simulink model "EngineBleedAirSystem"  (R2018b)
settings: Solver=FixedStepAuto  StartTime=0.0  StopTime=500  FixedStep=0.01  RelTol=1e-3
values from neighbouring files (symbols this model uses):
  AirSourceMode = 2    [run_sim.m]
libraries: simulink x2
settings Model: Creator=ZhaoJiance  LastModifiedBy=ZhaoJiance

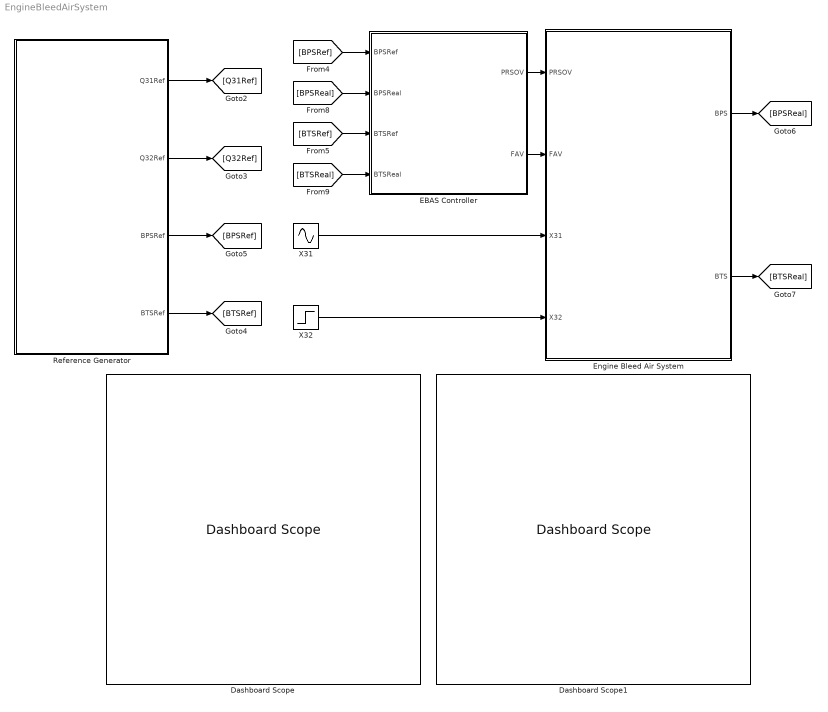
== system EngineBleedAirSystem ==
  Dashboard Scope : DashboardScope  WebBlockId=85
  Dashboard Scope1 : DashboardScope  WebBlockId=86
  EBAS Controller : Subsystem  VariantControlMode=Label  Variant=on  VariantControl=Variant1  LabelModeActiveChoice=L1AC
  Engine Bleed Air System : Subsystem
  Reference Generator : Subsystem
  X31 : Sin  Amplitude=10  Bias=50  Frequency=0.1  SampleTime=0
  X32 : Step  Time=0  Before=50  After=30  SampleTime=0
  wires:
  [BTSRef] -> EBAS Controller/3("BTSRef  ")
  [BPSReal] -> EBAS Controller/2("BPSReal ")
  EBAS Controller/2(" FAV") -> Engine Bleed Air System/2(FAV)
  Engine Bleed Air System/2(BTS) -> [BTSReal]
  Engine Bleed Air System/1(BPS) -> [BPSReal]
  EBAS Controller/1(" PRSOV") -> Engine Bleed Air System/1(PRSOV)
  [BPSRef] -> EBAS Controller/1("BPSRef  ")
  X31/1 -> Engine Bleed Air System/3(X31)
  [BTSReal] -> EBAS Controller/4("BTSReal  ")
  Reference Generator/4(BTSRef) -> [BTSRef]
  Reference Generator/2(Q32Ref) -> [Q32Ref]
  Reference Generator/1(Q31Ref) -> [Q31Ref]
  Reference Generator/3(BPSRef) -> [BPSRef]
  X32/1 -> Engine Bleed Air System/4(X32)

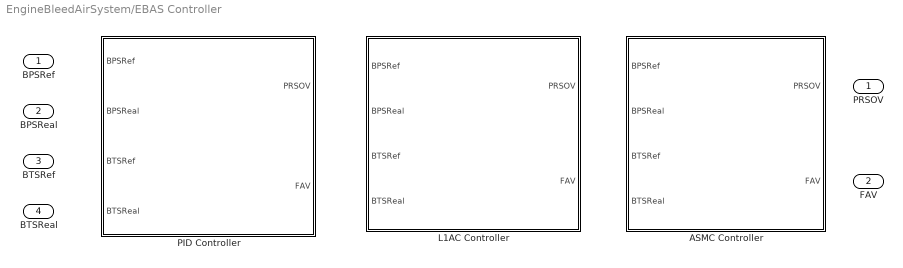
== system EngineBleedAirSystem/EBAS Controller ==
  "BPSRef  " : Inport
  "BPSReal " : Inport  Port=2
  "BTSRef  " : Inport  Port=3
  "BTSReal  " : Inport  Port=4
  ASMC Controller : Subsystem  VariantControl=ASMC
  L1AC Controller : Subsystem  VariantControl=L1AC
  PID Controller : Subsystem  VariantControl=PID
  " PRSOV" : Outport
  " FAV" : Outport  Port=2

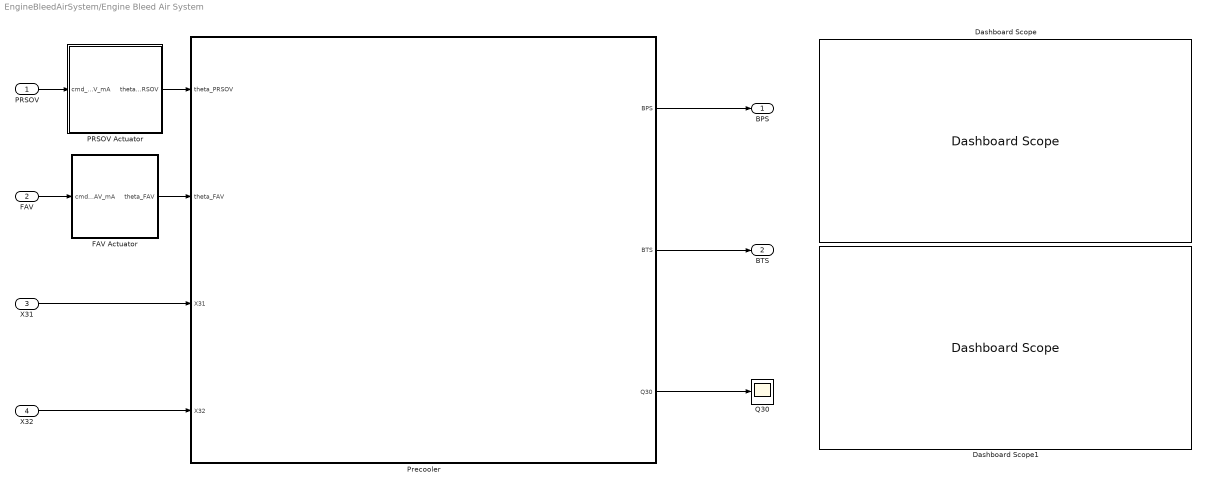
== system EngineBleedAirSystem/Engine Bleed Air System ==
  PRSOV : Inport
  FAV : Inport  Port=2
  X31 : Inport  Port=3
  X32 : Inport  Port=4
  Dashboard Scope : DashboardScope  WebBlockId=89
  Dashboard Scope1 : DashboardScope  WebBlockId=90
  FAV Actuator : MATLAB Function  TreatAsAtomicUnit=on  SystemSampleTime=0.01
  PRSOV Actuator : MATLAB Function  TreatAsAtomicUnit=on  SystemSampleTime=0.01
  Precooler : Subsystem
      mask Display: image('C:\Users\ZhaoJiance\Documents\Github\AeroBleedSimulation\SysID\figure\Precooler.png');
  Q30 : Scope
  BPS : Outport
  BTS : Outport  Port=2
  wires:
  FAV/1 -> FAV Actuator/1(cmd_FAV_mA)
  PRSOV/1 -> PRSOV Actuator/1(cmd_PRSOV_mA)
  PRSOV Actuator/1(theta_PRSOV) -> Precooler/1(theta_PRSOV)
  FAV Actuator/1(theta_FAV) -> Precooler/2(theta_FAV)
  Precooler/1(BPS) -> BPS/1
  Precooler/2(BTS) -> BTS/1
  Precooler/3(Q30) -> Q30/1
  X31/1 -> Precooler/3(X31)
  X32/1 -> Precooler/4(X32)

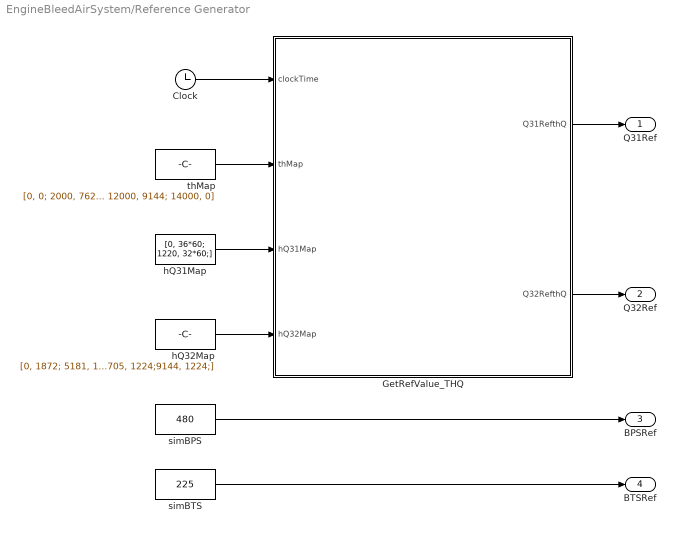
== system EngineBleedAirSystem/Reference Generator ==
  Clock : Clock
  GetRefValue_THQ : MATLAB Function  TreatAsAtomicUnit=on
  hQ31Map : Constant  Value=[0, 36*60; 1220, 32*60;]
  hQ32Map : Constant  Value=[0, 1872; 5181, 1872; 6705, 1224;9144, 1224;]
  simBPS : Constant  Value=480
  simBTS : Constant  Value=225
  thMap : Constant  Value=[0, 0; 2000, 7620; 4000, 7620;6000, 12192; 8000, 12192; 10000, 9144; 12000, 9144; 14000, 0]
  Q31Ref : Outport
  Q32Ref : Outport  Port=2
  BPSRef : Outport  Port=3
  BTSRef : Outport  Port=4
  wires:
  Clock/1 -> GetRefValue_THQ/1(clockTime)
  thMap/1 -> GetRefValue_THQ/2(thMap)
  hQ31Map/1 -> GetRefValue_THQ/3(hQ31Map)
  GetRefValue_THQ/1(Q31RefthQ) -> Q31Ref/1
  hQ32Map/1 -> GetRefValue_THQ/4(hQ32Map)
  GetRefValue_THQ/2(Q32RefthQ) -> Q32Ref/1
  simBTS/1 -> BTSRef/1
  simBPS/1 -> BPSRef/1

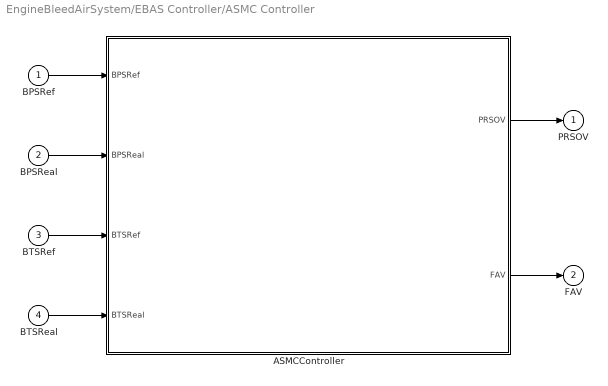
== system EngineBleedAirSystem/EBAS Controller/ASMC Controller ==
  "BPSRef  " : Inport
  "BPSReal " : Inport  Port=2
  "BTSRef  " : Inport  Port=3
  "BTSReal  " : Inport  Port=4
  ASMCController : MATLAB Function  TreatAsAtomicUnit=on  SystemSampleTime=0.01
  " PRSOV" : Outport
  " FAV" : Outport  Port=2
  wires:
  ASMCController/1(PRSOV) -> " PRSOV"/1
  ASMCController/2(FAV) -> " FAV"/1
  "BPSRef  "/1 -> ASMCController/1(BPSRef)
  "BPSReal "/1 -> ASMCController/2(BPSReal)
  "BTSRef  "/1 -> ASMCController/3(BTSRef)
  "BTSReal  "/1 -> ASMCController/4(BTSReal)

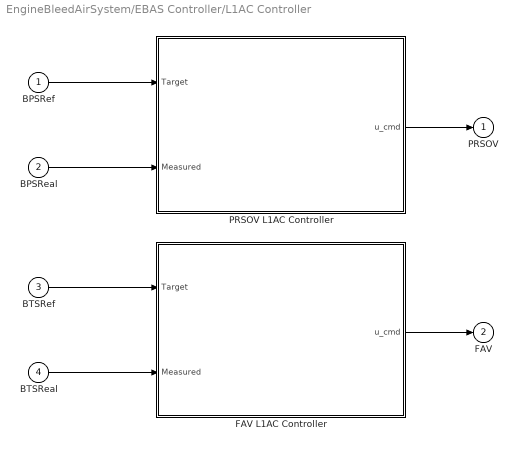
== system EngineBleedAirSystem/EBAS Controller/L1AC Controller ==
  "BPSRef  " : Inport
  "BPSReal " : Inport  Port=2
  "BTSRef  " : Inport  Port=3
  "BTSReal  " : Inport  Port=4
  FAV L1AC Controller : MATLAB Function  TreatAsAtomicUnit=on
  PRSOV L1AC Controller : MATLAB Function  TreatAsAtomicUnit=on
  " PRSOV" : Outport
  " FAV" : Outport  Port=2
  wires:
  FAV L1AC Controller/1(u_cmd) -> " FAV"/1
  PRSOV L1AC Controller/1(u_cmd) -> " PRSOV"/1
  "BPSRef  "/1 -> PRSOV L1AC Controller/1(Target)
  "BPSReal "/1 -> PRSOV L1AC Controller/2(Measured)
  "BTSReal  "/1 -> FAV L1AC Controller/2(Measured)
  "BTSRef  "/1 -> FAV L1AC Controller/1(Target)

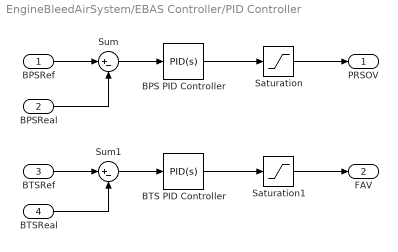
== system EngineBleedAirSystem/EBAS Controller/PID Controller ==
  "BPSRef " : Inport
  BPSReal : Inport  Port=2
  "BTSRef " : Inport  Port=3
  "BTSReal " : Inport  Port=4
  BPS PID Controller : simulink/Continuous/PID Controller  Controller=PID  Form=Parallel  TimeDomain=Continuous-time  SampleTime=-1  IntegratorMethod=Forward Euler  FilterMethod=Forward Euler  ControllerParametersSource=internal  P=0.1  I=0.2  D=0.01  UseFilter=on  N=100  TunerSelectOption=Transfer Function Based (PID Tuner App)  InitialConditionSource=internal  InitialConditionForIntegrator=0  InitialConditionForFilter=0  DifferentiatorICPrevScaledInput=0  ExternalReset=none  TrackingMode=off  Kt=1  LimitOutput=off  UpperSaturationLimit=inf  LowerSaturationLimit=-inf  LinearizeAsGain=on  AntiWindupMode=none  Kb=1  POutMin=[]  POutMax=[]  IOutMin=[]  IOutMax=[]  DOutMin=[]  DOutMax=[]  NOutMin=[]  NOutMax=[]  SumOutMin=[]  SumOutMax=[]  SaturationOutMin=[]  SaturationOutMax=[]  PParamMin=[]  PParamMax=[]  IParamMin=[]  IParamMax=[]  DParamMin=[]  DParamMax=[]  NParamMin=[]  NParamMax=[]  KbParamMin=[]  KbParamMax=[]  KtParamMin=[]  KtParamMax=[]  KbOutMin=[]  KbOutMax=[]  KtOutMin=[]  KtOutMax=[]  IntegratorOutMin=[]  IntegratorOutMax=[]  FilterOutMin=[]  FilterOutMax=[]  SumI1OutMin=[]  SumI1OutMax=[]  SumI2OutMin=[]  SumI2OutMax=[]  SumI3OutMin=[]  SumI3OutMax=[]  SumI4OutMin=[]  SumI4OutMax=[]  SumDOutMin=[]  SumDOutMax=[]  DifferentiatorOutMin=[]  DifferentiatorOutMax=[]  FilterDiffOutCoefMin=[]  FilterDiffOutCoefMax=[]  ReciprocalOutMin=[]  ReciprocalOutMax=[]  SumDenOutMin=[]  SumDenOutMax=[]  SumNumOutMin=[]  SumNumOutMax=[]  DivideOutMin=[]  DivideOutMax=[]  IntegratorContinuousStateAttributes=''  IntegratorStateMustResolveToSignalObject=off  IntegratorRTWStateStorageClass=Auto  FilterContinuousStateAttributes=''  FilterStateMustResolveToSignalObject=off  FilterRTWStateStorageClass=Auto  ParallelPVariant=InternalParameters  IdealPVariant=Disabled  IVariant=InternalParameters  DVariant=InternalParameters  IntegratorVariant=Continuous  SatVariant=Disabled  AWVariant=Passthrough  PCopyVariant=Disabled  TRVariant=Disabled  FdbkBlocksVariant=Forward  IdealPFdbkVariant=Disabled  SatFdbkVariant=Disabled  DerivativeFilterVariant=ContFilter  NVariant=InternalParameters  NCopyVariant=Disabled  FilterICVariant=InternalICsFilter  IntegratorICVariant=InternalICs  ExternalResetVariant=Disabled  TRSumVariant=Passthrough  SumFdbkVariant=Disabled  SumVariant=Sum_PID
  BTS PID Controller : simulink/Continuous/PID Controller  Controller=PID  Form=Parallel  TimeDomain=Continuous-time  SampleTime=-1  IntegratorMethod=Forward Euler  FilterMethod=Forward Euler  ControllerParametersSource=internal  P=-0.1  I=-0.15  D=0  UseFilter=on  N=100  TunerSelectOption=Transfer Function Based (PID Tuner App)  InitialConditionSource=internal  InitialConditionForIntegrator=0  InitialConditionForFilter=0  DifferentiatorICPrevScaledInput=0  ExternalReset=none  TrackingMode=off  Kt=1  LimitOutput=off  UpperSaturationLimit=inf  LowerSaturationLimit=-inf  LinearizeAsGain=on  AntiWindupMode=none  Kb=1  POutMin=[]  POutMax=[]  IOutMin=[]  IOutMax=[]  DOutMin=[]  DOutMax=[]  NOutMin=[]  NOutMax=[]  SumOutMin=[]  SumOutMax=[]  SaturationOutMin=[]  SaturationOutMax=[]  PParamMin=[]  PParamMax=[]  IParamMin=[]  IParamMax=[]  DParamMin=[]  DParamMax=[]  NParamMin=[]  NParamMax=[]  KbParamMin=[]  KbParamMax=[]  KtParamMin=[]  KtParamMax=[]  KbOutMin=[]  KbOutMax=[]  KtOutMin=[]  KtOutMax=[]  IntegratorOutMin=[]  IntegratorOutMax=[]  FilterOutMin=[]  FilterOutMax=[]  SumI1OutMin=[]  SumI1OutMax=[]  SumI2OutMin=[]  SumI2OutMax=[]  SumI3OutMin=[]  SumI3OutMax=[]  SumI4OutMin=[]  SumI4OutMax=[]  SumDOutMin=[]  SumDOutMax=[]  DifferentiatorOutMin=[]  DifferentiatorOutMax=[]  FilterDiffOutCoefMin=[]  FilterDiffOutCoefMax=[]  ReciprocalOutMin=[]  ReciprocalOutMax=[]  SumDenOutMin=[]  SumDenOutMax=[]  SumNumOutMin=[]  SumNumOutMax=[]  DivideOutMin=[]  DivideOutMax=[]  IntegratorContinuousStateAttributes=''  IntegratorStateMustResolveToSignalObject=off  IntegratorRTWStateStorageClass=Auto  FilterContinuousStateAttributes=''  FilterStateMustResolveToSignalObject=off  FilterRTWStateStorageClass=Auto  ParallelPVariant=InternalParameters  IdealPVariant=Disabled  IVariant=InternalParameters  DVariant=InternalParameters  IntegratorVariant=Continuous  SatVariant=Disabled  AWVariant=Passthrough  PCopyVariant=Disabled  TRVariant=Disabled  FdbkBlocksVariant=Forward  IdealPFdbkVariant=Disabled  SatFdbkVariant=Disabled  DerivativeFilterVariant=ContFilter  NVariant=InternalParameters  NCopyVariant=Disabled  FilterICVariant=InternalICsFilter  IntegratorICVariant=InternalICs  ExternalResetVariant=Disabled  TRSumVariant=Passthrough  SumFdbkVariant=Disabled  SumVariant=Sum_PID
  Saturation : Saturate  UpperLimit=400  LowerLimit=0
  Saturation1 : Saturate  UpperLimit=350  LowerLimit=0
  Sum : Sum  Inputs=|+-
  Sum1 : Sum  Inputs=|+-
  PRSOV : Outport
  FAV : Outport  Port=2
  wires:
  Sum1/1 -> BTS PID Controller/1
  BPS PID Controller/1 -> Saturation/1
  BTS PID Controller/1 -> Saturation1/1
  Sum/1 -> BPS PID Controller/1
  BPSReal/1 -> Sum/2
  "BPSRef "/1 -> Sum/1
  "BTSReal "/1 -> Sum1/2
  "BTSRef "/1 -> Sum1/1
  Saturation/1 -> PRSOV/1
  Saturation1/1 -> FAV/1

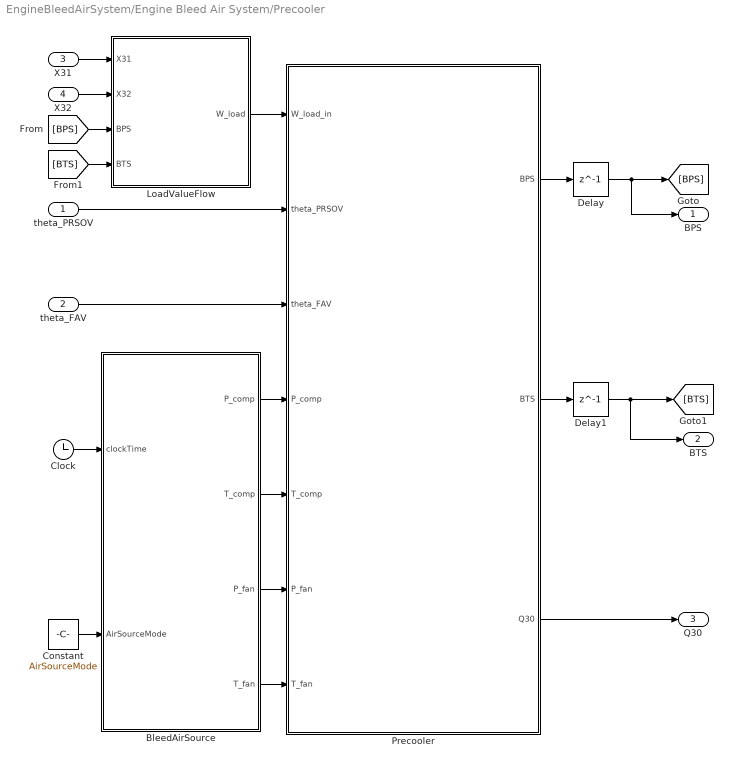
== system EngineBleedAirSystem/Engine Bleed Air System/Precooler ==
  theta_PRSOV : Inport
  theta_FAV : Inport  Port=2
  X31 : Inport  Port=3
  X32 : Inport  Port=4
  BleedAirSource : MATLAB Function  TreatAsAtomicUnit=on  SystemSampleTime=0.01
  Clock : Clock
  Constant : Constant  Value=AirSourceMode
  Delay : Delay  DelayLength=1  InitialCondition=0
  Delay1 : Delay  DelayLength=1  InitialCondition=0
  LoadValueFlow : MATLAB Function  TreatAsAtomicUnit=on  SystemSampleTime=0.01
  Precooler : MATLAB Function  TreatAsAtomicUnit=on  SystemSampleTime=0.01
  BPS : Outport
  BTS : Outport  Port=2
  Q30 : Outport  Port=3
  wires:
  Delay/1 -> BPS/1, [BPS]
  Delay1/1 -> BTS/1, [BTS]
  LoadValueFlow/1(W_load) -> Precooler/1(W_load_in)
  Precooler/1(BPS) -> Delay/1
  Precooler/2(BTS) -> Delay1/1
  Precooler/3(Q30) -> Q30/1
  theta_PRSOV/1 -> Precooler/2(theta_PRSOV)
  theta_FAV/1 -> Precooler/3(theta_FAV)
  X31/1 -> LoadValueFlow/1(X31)
  X32/1 -> LoadValueFlow/2(X32)
  Clock/1 -> BleedAirSource/1(clockTime)
  [BTS] -> LoadValueFlow/4(BTS)
  [BPS] -> LoadValueFlow/3(BPS)
  BleedAirSource/1(P_comp) -> Precooler/4(P_comp)
  BleedAirSource/2(T_comp) -> Precooler/5(T_comp)
  BleedAirSource/3(P_fan) -> Precooler/6(P_fan)
  BleedAirSource/4(T_fan) -> Precooler/7(T_fan)
  Constant/1 -> BleedAirSource/2(AirSourceMode)

== matlab function EngineBleedAirSystem/EBAS Controller/ASMC Controller/ASMCController ==
  data: BPSRef input; PRSOV output; BPSReal input; BTSRef input; BTSReal input; FAV output
function [PRSOV, FAV] = ASMCController(BPSRef, BPSReal, BTSRef, BTSReal)
    % =========================================================================
    % 引气系统控制器 (ESO + ASMC + 逆迟滞补偿)
    %
    % 架构说明:
    %   1. 观测层 (ESO): 实时估计系统内部状态和未知负载扰动(Total Disturbance)。
    %   2. 决策层 (ASMC): 基于扰动补偿的自适应滑模控制，计算理想阀门角度。
    %   3. 补偿层 (Inverse Hys): 将理想角度映射为电流，抵消物理迟滞。
    %
    % 输入:
    %   BPSRef/Real : 压力期望/反馈 [kPa]
    %   BTSRef/Real : 温度期望/反馈 [degC]
    % 输出:
    %   PRSOV    : 热路阀电流 [0-400mA]
    %   FAV      : 冷路阀电流 [0-350mA]
    % =========================================================================

    % --- 1. 系统参数与状态存储 ---
    persistent z1_p z2_p        % 压力ESO状态: z1(压力估计), z2(总扰动)
    persistent z1_t z2_t        % 温度ESO状态: z1(温度估计), z2(总扰动)
    persistent k_asmc_p         % 压力控制器自适应增益
    persistent k_asmc_t         % 温度控制器自适应增益
    persistent last_theta_p     % 上一时刻压力阀角度(用于判断方向)
    persistent last_theta_f     % 上一时刻温度阀角度
    persistent is_init          % 初始化标志

    % --- 2. 参数初始化 ---
    if isempty(is_init)
        % ESO 初始状态
        z1_p = BPSReal; z2_p = 0;
        z1_t = BTSReal; z2_t = 0;
        
        % ASMC 初始增益
        k_asmc_p = 5.0; 
        k_asmc_t = 2.0;
        
        last_theta_p = 0;
        last_theta_f = 0;
        is_init = 1;
    end
    
    dt = 0.01; % 采样时间 [s]

    % =====================================================================
    % 3. 压力控制回路 (Pressure Control Loop)
    %    目标: BPS -> BPSRef
    %    策略: ESO 估计负载扰动 -> ASMC 计算角度 -> 逆模型输出电流
    % =====================================================================
    
    % --- 3.1 扩张状态观测器 (ESO) ---
    % 标称控制增益 b0_p (估算值: 阀门对压力的影响率)
    % 物理意义: 开度增加1度，压力大约增加多少kPa/s
    b0_p = 20.0; 
    
    % ESO 参数 (带宽配置)
    beta1_p = 100; % 状态观测增益
    beta2_p = 100; % 扰动观测增益
    
    % 观测器误差
    e_eso_p = z1_p - BPSReal;
    
    % ESO 状态更新 (离散化欧拉法)
    % u_last 近似为上一时刻的角度 last_theta_p
    dz1_p = z2_p + b0_p * (last_theta_p/90.0) - beta1_p * e_eso_p;
    dz2_p = -beta2_p * e_eso_p;
    
    z1_p = z1_p + dz1_p * dt;
    z2_p = z2_p + dz2_p * dt;
    
    % z2_p 即为估计出的"总扰动" (包含 X31/X32 动作引起的压力跌落)
    
    % --- 3.2 自适应滑模控制器 (ASMC) ---
    e_p = BPSRef - BPSReal; % 跟踪误差
    
    % 自适应律: 根据误差大小调整增益
    % 误差大 -> 增益增大; 误差小 -> 增益保持
    eta_p = 2.0;
    dk_p = eta_p * abs(e_p);
    k_asmc_p = min(max(k_asmc_p + dk_p * dt, 1.0), 50.0); % 增益限幅
    
    % 控制律计算
    % u = (1/b0) * (dot_ref - z2 + k * tanh(s))
    % 这里忽略 dot_ref (假设阶跃输入)，引入 tanh 平滑切换
    phi_p = 25.0; % 边界层厚度
    u_ideal_p_norm = (1/b0_p) * (-z2_p + k_asmc_p * tanh(e_p/phi_p));
    
    % 反归一化到角度 [0, 90]
    theta_p_des = u_ideal_p_norm * 90.0;
    theta_p_des = max(0, min(90, theta_p_des)); % 物理限幅
    
    % --- 3.3 迟滞补偿 (逆模型层) ---
    % 使用查表法代替神经网络 (功能等效: 映射 理想角度 -> 实际电流)
    I_axis_P = [0, 120.0, 137.5, 155.0, 172.5, 190.0, 225.0, 260.0, 295.0, 330.0, 365.0, 400.0];
    
    Ang_Rise_P = [-1.0, 0, 3, 7, 15, 25, 45, 62, 75, 85, 89, 90]; 
    Ang_Fall_P = [-1.0, 0, 10, 25, 40, 55, 75, 85, 89, 90, 90.1, 90.2];
    
    % 判断运动方向
    if theta_p_des >= last_theta_p
        PRSOV = interp1(Ang_Rise_P, I_axis_P, theta_p_des, 'linear', 'extrap');
    else
        PRSOV = interp1(Ang_Fall_P, I_axis_P, theta_p_des, 'linear', 'extrap');
    end
    PRSOV = max(0, min(400, PRSOV));
    
    % =====================================================================
    % 4. 温度控制回路 (Temperature Control Loop)
    %    目标: BTS -> BTSRef
    %    注意: 这是一个反向响应系统 (开大冷风阀 -> 温度降低)
    % =====================================================================
    
    % --- 4.1 ESO ---
    b0_t = -10.0; % 负增益: 角度增加，温度下降
    beta1_t = 50; 
    beta2_t = 200;
    
    e_eso_t = z1_t - BTSReal;
    dz1_t = z2_t + b0_t * (last_theta_f/90.0) - beta1_t * e_eso_t;
    dz2_t = -beta2_t * e_eso_t;
    
    z1_t = z1_t + dz1_t * dt;
    z2_t = z2_t + dz2_t * dt;
    
    % --- 4.2 ASMC ---
    e_t = BTSRef - BTSReal;
    
    eta_t = 1.0;
    dk_t = eta_t * abs(e_t);
    k_asmc_t = min(max(k_asmc_t + dk_t * dt, 1.0), 30.0);
    
    % 控制律 (注意 b0_t 是负数，会自动处理方向)
    phi_t = 30;
    u_ideal_t_norm = (1/b0_t) * (-z2_t + k_asmc_t * tanh(e_t/phi_t));
    
    theta_f_des = u_ideal_t_norm * 90.0;
    theta_f_des = max(0, min(90, theta_f_des));
    
    % --- 4.3 迟滞补偿 ---
    I_axis_F = [0, 120.0000, 134.3750, 148.7500, 163.1250, 177.5000, ...
                206.2500, 235.0000, 263.7500, 292.5000, 321.2500, 350.0000];
    
    Ang_Rise_F = [-1.0, 0, 3, 7, 15, 25, 45, 62, 75, 85, 89, 90]; 
    Ang_Fall_F = [-1.0, 0, 10, 25, 40, 55, 75, 85, 89, 90, 90.1, 90.2];
    
    if theta_f_des >= last_theta_f
        FAV = interp1(Ang_Rise_F, I_axis_F, theta_f_des, 'linear', 'extrap');
    else
        FAV = interp1(Ang_Fall_F, I_axis_F, theta_f_des, 'linear', 'extrap');
    end
    FAV = max(0, min(350, FAV));
    
    % =====================================================================
    % 5. 状态更新
    % =====================================================================
    last_theta_p = theta_p_des;
    last_theta_f = theta_f_des;

end

== matlab function EngineBleedAirSystem/Engine Bleed Air System/Precooler/LoadValueFlow ==
  data: X31 input; W_load output; X32 input; BPS input; BTS input
function W_load = LoadValueFlow(X31, X32, BPS, BTS)
    % =========================================================================
    % LoadValveFlow: 下游双管路负载流量计算模块
    %
    % --- 修正说明 ---
    % 1. 修复了温度计算错误：输入的 BTS 是摄氏度，必须转为开尔文计算流量。
    % 2. 修正了注释，明确需要 4 个输入。
    %
    % --- 输入 (Inputs) ---
    % 1. X31    : 下游管路31空调路 阀门开度指令 [%] (0~100)
    % 2. X32    : 下游管路32防冰路 阀门开度指令 [%] (0~100)
    % 3. BPS    : 上游压力 (即 Precooler 输出的 BPS) [kPa]
    % 4. BTS    : 上游温度 (即 Precooler 输出的 BTS) [degC]
    %
    % --- 输出 (Outputs) ---
    % 1. W_load : 总排气流量 [kg/h]
    % =========================================================================

    % --- 物理常数 ---
    R = 287.05;       
    Gamma = 1.4;      
    P_amb_Pa = 101325; 
    
    % --- 单位转换 ---
    Pup_load = BPS * 1000;        % [kPa] -> [Pa]
    T_up_K   = BTS + 273.15;      % [degC] -> [K]
    
    % --- 计算总流通面积 ---
    D_load = 0.1;   % DN100 [m]
    Cd_load = 0.8;  
    A_max_single = pi * D_load^2 / 4;

    ratio1 = max(min(X31, 100), 0) / 100;
    ratio2 = max(min(X32, 100), 0) / 100;
    
    A1 = Cd_load * A_max_single * ratio1;
    A2 = Cd_load * A_max_single * ratio2;
    A_load_total = A1 + A2;
    
    % --- 计算流量 ---
    Pdn_load = P_amb_Pa;     
    
    % 只有当上游压力大于环境压力，且阀门有开度时才计算
    % 增加 T_up_K > 0 保护，防止仿真初期温度异常导致 sqrt 报错
    if Pup_load > Pdn_load && A_load_total > 1e-6 && T_up_K > 0
        pr_load = Pdn_load / Pup_load;
        
        if pr_load < 0.528
            Psi_load = sqrt(Gamma * (2/(Gamma+1))^((Gamma+1)/(Gamma-1)));
        else
            Psi_load = sqrt(2*Gamma/(Gamma-1) * (pr_load^(2/Gamma) - pr_load^((Gamma+1)/Gamma)));
        end
        
        % 使用开尔文温度 T_up_K 进行计算
        W_load_kgs = A_load_total * (Pup_load / sqrt(R * T_up_K)) * Psi_load;
        
        W_load = W_load_kgs * 3600;
    else
        W_load = 0;
    end
end

== matlab function EngineBleedAirSystem/Reference Generator/GetRefValue_THQ ==
  data: clockTime input; thMap input; hQ31Map input; hQ32Map input; Q31RefthQ output; Q32RefthQ output
function [Q31RefthQ, Q32RefthQ] = getRefValue_THQ(clockTime, thMap, hQ31Map, hQ32Map)
    elapsedTime = max(min(clockTime, max(thMap(:,1))), min(thMap(:,1)));
    
    % 排序 + 去重（按高度第一列）
    thMap   = sortrows(thMap, 1);    [~, idx_th] = unique(thMap(:,1), 'stable'); thMap = thMap(idx_th, :);
    hQ31Map = sortrows(hQ31Map, 1);  [~, idx31] = unique(hQ31Map(:,1), 'stable'); hQ31Map = hQ31Map(idx31, :);
    hQ32Map = sortrows(hQ32Map, 1);  [~, idx32] = unique(hQ32Map(:,1), 'stable'); hQ32Map = hQ32Map(idx32, :);

    % 计算当前高度（时间 → 高度）
    currentHeight = interp1(thMap(:,1), thMap(:,2), elapsedTime, 'linear', 'extrap');

    % 获取各流量的最小和最大高度
    minHeight_Q31 = min(hQ31Map(:,1)); maxHeight_Q31 = max(hQ31Map(:,1));
    minHeight_Q32 = min(hQ32Map(:,1)); maxHeight_Q32 = max(hQ32Map(:,1));

    % 限制 currentHeight 在各自的高度范围内
    height_Q31 = min(max(currentHeight, minHeight_Q31), maxHeight_Q31);
    height_Q32 = min(max(currentHeight, minHeight_Q32), maxHeight_Q32);

    % 计算各个流量值（高度 → 流量）
    Q31RefthQ = interp1(hQ31Map(:,1), hQ31Map(:,2), height_Q31, 'linear', 'extrap');
    Q32RefthQ = interp1(hQ32Map(:,1), hQ32Map(:,2), height_Q32, 'linear', 'extrap');
end

== matlab function EngineBleedAirSystem/Engine Bleed Air System/Precooler/Precooler ==
  data: W_load_in input; theta_PRSOV input; BPS output; theta_FAV input; P_comp input; BTS output; Q30 output; T_comp input; P_fan input; T_fan input
function [BPS, BTS, Q30] = Precooler(W_load_in, theta_PRSOV, theta_FAV, P_comp, T_comp, P_fan, T_fan)
    % =========================================================================
    % Precooler Integrated Plant Model
    %
    % --- 输入 (Inputs) ---
    % 1. theta_PRSOV : 压力调节关断阀(PRSOV)开度角度 [deg] (0~90)
    % 2. T_comp      : 压气机引气温度 [degC]
    % 3. P_fan       : 风扇流路压力 [kPa]
    % 4. T_fan       : 风扇流路温度 [degC]
    % 5. theta_FAV   : 风扇空气阀(FAV)开度角度 [deg] (0~90)
    % 6. P_comp      : 压气机引气压力 [kPa]
    % 7. W_load_in   : 外部输入的下游负载流量 [kg/h] 
    %                  (由 LoadValveFlow 函数计算得出)
    %
    % --- 输出 (Outputs) ---
    % 1. BPS         : 预冷器热路出口压力 (Bleed Pressure Sensor) [kPa]
    % 2. BTS         : 预冷器热路出口温度 (Bleed Temperature Sensor) [degC]
    % 3. Q30         : 预冷器热路出口引气流量 [kg/h]
    % =========================================================================

    % --- 状态变量声明 ---
    % P_store: 下游管路容腔压力 [Pa]
    % T_store: 下游管路容腔温度 [K] (混合后的最终温度)
    % T_hx_out: 预冷器芯体出口温度 [K] (新增状态，体现换热器本身的热惯性)
    persistent P_store T_store T_hx_out
    
    % --- 仿真参数 ---
    dt = 0.01; % 固定时间步长 [s]
    
    % 物理常数
    R = 287.05;       
    Gamma = 1.4;      
    P_amb_Pa = 101325;
    
    % 下游容积计算
    % 2个管路，每个均为 DN100，长度 5m
    Vol = 2 * (pi * 0.05^2 * 5);          
    
    % --- 初始化 ---
    if isempty(P_store)
        P_store = P_amb_Pa;         % 初始为环境压力
        T_store = T_comp + 273.15;  % 初始温度
        T_hx_out = T_comp + 273.15; 
    end
    
    % 单位转换
    P_comp_Pa = P_comp * 1000;       
    T_comp_K  = T_comp + 273.15;
    P_fan_Pa  = P_fan * 1000;        
    T_fan_K   = T_fan + 273.15;        
    
    % =====================================================================
    % 1. 进气流量计算 (Source Flow)
    % =====================================================================
    
    % --- 热路入口阀 (PRSOV) ---
    D_prsov = 0.1;    
    Cd_prsov = 0.8;   
    phi_p = theta_PRSOV * (pi/180); 
    A_prsov = Cd_prsov * (pi * D_prsov^2 / 4) * (1 - cos(phi_p));
    
     % 判断流向
    if P_comp_Pa >= P_store
        Pup = P_comp_Pa; Pdn = P_store; T_up = T_comp_K; Is_Reverse = 1;
    else
        Pup = P_store; Pdn = P_comp_Pa; T_up = T_store; Is_Reverse = -1;
    end
    
    % 计算流量 (圣维南公式)
    if Pup > 1 && A_prsov > 1e-6
        pr = Pdn / Pup; 
        if pr > 1, pr = 1; end 
        if pr < 0, pr = 0; end

        pr_crit = 0.528; 
        if pr < pr_crit
            Psi = sqrt(Gamma * (2/(Gamma+1))^((Gamma+1)/(Gamma-1))); 
        else
            Psi = sqrt(2*Gamma/(Gamma-1) * (pr^(2/Gamma) - pr^((Gamma+1)/Gamma)));
        end
        W_bleed = A_prsov * (Pup / sqrt(R * T_up)) * Psi * Is_Reverse;
    else
        W_bleed = 0;
    end
    
    Q30 = W_bleed * 3600; 

    % =====================================================================
    % 2. 冷却气流计算 (Cooling Flow)
    % =====================================================================
    D_fav = 0.14;     
    Cd_fav = 0.8;     
    phi_f = theta_FAV * (pi/180);
    A_fav = Cd_fav * (pi * D_fav^2 / 4) * (1 - cos(phi_f));
    
    if P_fan_Pa > P_amb_Pa && A_fav > 0
        ratio = P_amb_Pa / P_fan_Pa;
        if ratio > 0.528
            Psi_f = sqrt(2*Gamma/((Gamma-1)*R*T_fan_K) * (ratio^(2/Gamma) - ratio^((Gamma+1)/Gamma)));
        else
            Psi_f = sqrt(2*Gamma/((Gamma-1)*R*T_fan_K) * (0.528^(2/Gamma) - 0.528^((Gamma+1)/Gamma)));
        end
        W_fan = A_fav * P_fan_Pa * Psi_f;
    else
        W_fan = 0;
    end
    
    % =====================================================================
    % 3. 换热机理修正
    % 参考文献[1]: 石周正, 等. 飞行器引气系统预冷器动态模型搭建及辨识研究[J]. 
    %          西北工业大学学报, 2024, 42(6): 1089-1098.
    %   1. 引入了论文中的"变时间常数"热惯性机理 (Eq. 14)。
    %   2. 将瞬态换热改为一阶动态响应过程，更符合物理实测。
    % =====================================================================
    
    % 3.1 计算稳态目标温度 (Steady State Target)
    % 这是假设时间无限长后应该达到的温度
    if abs(W_bleed) > 1e-4
        flow_ratio = W_fan / abs(W_bleed);
        
        % 效率曲线
        % 参考文献[2]: 卜绍志.飞机引气系统温度控制研究[J].内燃机与配件,2025,(13):52-54.
        x_d = [0, 0.26, 0.76, 1.26, 1.76, 2.26, 2.76, 3.26, 4.0, 5.0];
        y_d = [0, 0.32, 0.65, 0.78, 0.85, 0.89, 0.92, 0.94, 0.96, 0.97];
        
        % 限制输入范围，防止超出插值表
        flow_ratio_clamped = min(max(flow_ratio, 0), 5.0);
        eta = interp1(x_d, y_d, flow_ratio_clamped, 'linear');
        
        T_target = T_comp_K - eta * (T_comp_K - T_fan_K);
        
        
        % 3.2 计算流速与时间常数 (参考文献[1] Eq. 14)
        % 估算流经预冷器芯体的热路流速 v_h [m/s]
        % 假设芯体有效流通面积 A_core (需根据预冷器尺寸估算，例如 0.005 m^2)
        A_core = 0.005; 
        % 密度 rho = P / (R * T)
        rho_h = Pup / (R * T_up);
        v_h = abs(W_bleed) / (rho_h * A_core);
        
        % 防止 v_h 过小导致除零或时间常数过大
        v_h = max(v_h, 0.5); 
        
        % 参考文献[1] Eq. 14: tau = 38.02 * v^(-0.394)
        % 系数 38.02 是论文针对特定型号辨识的，可作为通用参考
        tau_hx = 38.02 * (v_h ^ -0.394);
        
        % 限制时间常数范围 (例如 0.1s 到 10s)
        tau_hx = max(min(tau_hx, 10), 0.1);
        
        % 2.3 换热器热惯性动态更新 (一阶滞后)
        % dT_hx/dt = (T_target - T_hx_out) / tau
        dT_hx = (T_target - T_hx_out) / tau_hx * dt;
        T_hx_out = T_hx_out + dT_hx;
        
    else
        % 无流量时，温度趋向于环境或保持不变
        % 这里简化为缓慢趋向于环境温度 (自然冷却)
        tau_cooling = 20.0; % 较慢的自然冷却
        dT_hx = (T_comp_K - T_hx_out) / tau_cooling * dt; 
        T_hx_out = T_hx_out + dT_hx;
    end
    
    % =====================================================================
    % 4. 容腔动态积分 (Chamber Integration)
    % =====================================================================
    
    % 直接使用外部输入的 W_load_in
    % W_load_in 必须为正值 (流出)
    % 输入单位是 [kg/h]，物理计算需要 [kg/s]，所以除以 3600
    W_load = abs(W_load_in) / 3600.0;
    
    % 4.1 压力积分
    dP = (R * T_store / Vol) * (W_bleed - W_load) * dt;

    P_new = P_store + dP;
    if P_new < P_amb_Pa
        P_new = P_amb_Pa;
    end
    
    % 4.2 温度积分
    Current_Mass = P_store * Vol / (R * T_store);
    if Current_Mass < 1e-4; Current_Mass = 1e-4; end
    
    if W_bleed > 0
        % 正向流：T_hx_out 进入容腔与 T_store 混合
        dT_chamber = (1/Current_Mass) * (W_bleed * (T_hx_out - T_store)) * dt;
    else
        % 反向流或无流：温度缓慢恢复到环境或保持
        dT_chamber = -0.01 * (T_store - 293.15) * dt;
    end
    
    T_new = T_store + dT_chamber;
    
    % 更新状态
    P_store = P_new;
    T_store = T_new;
    
    % 输出赋值
    BPS = P_store / 1000;           
    BTS = T_store - 273.15;   
end

== matlab function EngineBleedAirSystem/Engine Bleed Air System/Precooler/BleedAirSource ==
  data: clockTime input; P_comp output; T_comp output; P_fan output; T_fan output; AirSourceMode input
function [P_comp, T_comp, P_fan, T_fan] = BleedAirSource(clockTime, AirSourceMode)
    % =========================================================================
    % 飞机环境与引气参数模拟源
    %
    % 输入: 
    %   clockTime : 仿真时间 [s]
    %   AirSourceMode   : 仿真模式选择
    %                       1 = 动态任务剖面 (Dynamic Mission Profile)
    %                       2 = 静态设计点 (Static Design Point)
    %                       3 = 静态设计点 + 正弦波动 (Static + Sine Wave)
    % 输出: 
    %   P_comp: 热路引气压力 [kPa]
    %   T_comp: 热路引气温度 [degC]
    %   P_fan : 冷路风扇压力 [kPa]
    %   T_fan : 冷路风扇温度 [degC]
    % =========================================================================

    if AirSourceMode == 1
        % =================================================================
        % 模式 1: 动态飞行任务剖面 (随时间变化)
        % =================================================================
        
        % 1. 定义飞行剖面节点 [时间(s), 高度(m)]
        t_points = [0,    2000, 4000, 6000,  8000,  10000, 12000, 14000];
        h_points = [0,    7620, 7620, 12192, 12192, 9144,  9144, 0];
        
        t_safe = max(min(clockTime, 14000), 0); % 限制时间范围
        
        % 2. 计算当前高度 (线性插值)
        Alt = interp1(t_points, h_points, t_safe, 'linear');
        
        % 3. 计算国际标准大气 (ISA)
        % 温度递减率: -6.5 C/km
        % 海平面: 15 C, 101.325 kPa
        T_amb_C = 15 - 0.0065 * Alt;
        T_amb_K = T_amb_C + 273.15;
        % 压力高度公式 (对流层)
        P_amb_kPa = 101.325 * (1 - 2.25577e-5 * Alt)^5.2559;
        
        % 4. 发动机参数解算
        Gamma = 1.4;
        
        % --- 冷路 (Fan) ---
        FPR = 1.6; % 风扇压比
        P_fan = P_amb_kPa * FPR;
        % 绝热压缩温升
        T_fan_K = T_amb_K * (FPR^((Gamma-1)/Gamma));
        T_fan = T_fan_K - 273.15;        % 输出摄氏度
        
        % --- 热路 (Compressor) ---
        CPR = 12; % 压气机压比
        eff = 0.85; % 绝热效率
        P_comp = P_amb_kPa * CPR;
        % 压气机出口温度计算
        T_comp_K = T_amb_K * (1 + (CPR^((Gamma-1)/Gamma) - 1) / eff);
        T_comp = T_comp_K - 273.15; % 输出摄氏度
        
    elseif AirSourceMode == 2
        % =================================================================
        % 模式 2: 静态设计点 (常值)
        % 适用于PID参数整定或稳态特性研究
        % =================================================================
        
        % 热路设定 (典型高压引气)
        P_comp = 600;   % [kPa]
        T_comp = 280;   % [degC]
        
        % 冷路设定 (典型地面或低空风扇出口)
        P_fan  = 110;   % [kPa]
        T_fan  = 30;    % [degC]

    elseif AirSourceMode == 3
        % =================================================================
        % 模式 3: 静态设计点 + 正弦波动干扰
        % 适用于测试控制系统的抗干扰能力和动态调节性能
        % =================================================================

        % --- 基础静态值 (与模式2相同) ---
        Base_P_comp = 600;
        Base_T_comp = 280;
        Base_P_fan  = 110;
        Base_T_fan  = 30;

        % --- 波动参数设置 ---
        % 频率 Hz (0.01 Hz = 100秒一个周期)
        Freq_P = 0.01; 
        Freq_T = 0.005; % 温度变化通常比压力慢，设为更低频率

        % 振幅 (波动的大小)
        Amp_P_comp = 20;  % 压力波动 +/- 50 kPa
        Amp_T_comp = 5;  % 温度波动 +/- 5 degC
        Amp_P_fan  = 5;  % 风扇压力波动较小
        Amp_T_fan  = 5;   

        % --- 计算波动值 ---
        % 公式: Base + Amplitude * sin(2 * pi * f * t)
        P_comp = Base_P_comp + Amp_P_comp * sin(2 * pi * Freq_P * clockTime);
        T_comp = Base_T_comp + Amp_T_comp * sin(2 * pi * Freq_T * clockTime);
        
        P_fan  = Base_P_fan  + Amp_P_fan  * sin(2 * pi * Freq_P * clockTime);
        T_fan  = Base_T_fan  + Amp_T_fan  * sin(2 * pi * Freq_T * clockTime);

    else
        % 默认防错输出
        P_comp = 101.3;
        T_comp = 15;
        P_fan = 101.3;
        T_fan = 15;
    end

end

== matlab function EngineBleedAirSystem/EBAS Controller/L1AC Controller/PRSOV L1AC Controller ==
  data: Target input; u_cmd output; Measured input; P_L1 parameter
function u_cmd = L1_Controller(Target, Measured, P_L1)
    % =========================================================================
    % L1 Adaptive Controller (Discrete Time Implementation)
    % 
    % Inputs:
    %   Target   - 设定值 (如目标压力 480kPa 或目标温度 200C)
    %   Measured - 实际测量值
    %   Am       - 参考模型带宽 (期望的系统响应速度, >0)
    %   Gamma    - 自适应增益 (学习率, 越大收敛越快但可能震荡)
    %   Bm       - 标称控制增益 (估算的系统输入效能 B矩阵)
    %   Wc       - L1滤波器截止频率 (决定了控制器的频带宽度)
    %
    % Output:
    %   u_cmd    - 控制指令 (0~1)
    % =========================================================================
    
    Am = P_L1.Press.Am;
    Gamma = P_L1.Press.Gamma;
    Bm = P_L1.Press.Bm;
    Wc = P_L1.Press.Wc;

    % --- 状态记忆 ---
    persistent x_hat      % 状态观测值 (Predictor State)
    persistent sigma_hat  % 扰动/不确定性估计值 (Adaptive Estimate)
    persistent u_filter   % 经过滤波后的控制量 (Filtered Control)
    
    % --- 采样时间 ---
    % 必须与 Simulink Solver 的 Fixed-step size 保持一致
    dt = 0.01; 
    
    % --- 初始化 ---
    if isempty(x_hat)
        x_hat = Measured; % 初始观测值跟随测量值
        sigma_hat = 0;
        u_filter = 0;     % 假设初始阀门关闭或处于某个中间值
    end
    
    % =====================================================================
    % 1. 状态预测器 (State Predictor)
    %    理论模型: x_dot_hat = -Am * x_hat + Bm * u + sigma_hat
    %    x_hat 试图追踪真实的 Measured 值，两者的差异驱动自适应律
    % =====================================================================
    % 使用上一时刻的控制量 u_filter 进行预测
    x_hat_dot = -Am * x_hat + Bm * u_filter + sigma_hat;
    
    % 欧拉积分更新预测状态
    x_hat_next = x_hat + x_hat_dot * dt;
    
    % =====================================================================
    % 2. 误差计算 (Prediction Error)
    %    x_tilde = x_hat - x_real
    % =====================================================================
    x_tilde = x_hat - Measured;
    
    % =====================================================================
    % 3. 自适应律 (Adaptation Law)
    %    sigma_dot_hat = -Gamma * x_tilde
    %    基于 Lyapunov 稳定性推导，用于快速估计总扰动 sigma
    % =====================================================================
    sigma_dot = -Gamma * x_tilde;
    
    % 更新扰动估计
    sigma_hat_next = sigma_hat + sigma_dot * dt;
    
    % =====================================================================
    % 4. 控制律计算 (Control Law)
    %    目标: 消除扰动 sigma 并跟踪参考信号 Target
    %    u_raw = (Am * Target - sigma_hat) / Bm
    %    (这里假设我们希望闭环系统行为像 dx/dt = -Am*x + Am*Target)
    % =====================================================================
    u_raw = (Am * Target - sigma_hat_next) / Bm;
    
    % =====================================================================
    % 5. 低通滤波器 (Low-Pass Filter) - L1 控制器的关键特征
    %    C(s) = Wc / (s + Wc)
    %    过滤掉高频自适应噪声，仅让低频有效控制信号通过
    % =====================================================================
    u_dot = -Wc * u_filter + Wc * u_raw;
    u_filter_next = u_filter + u_dot * dt;
    
    % =====================================================================
    % 6. 输出限幅与状态更新
    % =====================================================================
    % 物理执行机构限制 (0 ~ 1)
    u_cmd = max(min(u_filter_next, 1), 0);
    
    % 更新 Persistent 变量供下一次计算使用
    x_hat = x_hat_next;
    sigma_hat = sigma_hat_next;
    
    % 注意：这里使用限幅后的 u_cmd 更新 u_filter，
    % 可以在一定程度上防止积分器(滤波器)饱和 (Anti-windup 效应)
    u_filter = u_cmd; 
end

== matlab function EngineBleedAirSystem/EBAS Controller/L1AC Controller/FAV L1AC Controller ==
  data: Target input; u_cmd output; Measured input; P_L1 parameter
function u_cmd = L1_Controller(Target, Measured, P_L1)
    % =========================================================================
    % L1 Adaptive Controller (Discrete Time Implementation)
    % 
    % Inputs:
    %   Target   - 设定值 (如目标压力 480kPa 或目标温度 200C)
    %   Measured - 实际测量值
    %   Am       - 参考模型带宽 (期望的系统响应速度, >0)
    %   Gamma    - 自适应增益 (学习率, 越大收敛越快但可能震荡)
    %   Bm       - 标称控制增益 (估算的系统输入效能 B矩阵)
    %   Wc       - L1滤波器截止频率 (决定了控制器的频带宽度)
    %
    % Output:
    %   u_cmd    - 控制指令 (0~1)
    % =========================================================================
    
    Am = P_L1.Temp.Am;
    Gamma = P_L1.Temp.Gamma;
    Bm = P_L1.Temp.Bm;
    Wc = P_L1.Temp.Wc;

    % --- 状态记忆 ---
    persistent x_hat      % 状态观测值 (Predictor State)
    persistent sigma_hat  % 扰动/不确定性估计值 (Adaptive Estimate)
    persistent u_filter   % 经过滤波后的控制量 (Filtered Control)
    
    % --- 采样时间 ---
    % 必须与 Simulink Solver 的 Fixed-step size 保持一致
    dt = 0.01; 
    
    % --- 初始化 ---
    if isempty(x_hat)
        x_hat = Measured; % 初始观测值跟随测量值
        sigma_hat = 0;
        u_filter = 0;     % 假设初始阀门关闭或处于某个中间值
    end
    
    % =====================================================================
    % 1. 状态预测器 (State Predictor)
    %    理论模型: x_dot_hat = -Am * x_hat + Bm * u + sigma_hat
    %    x_hat 试图追踪真实的 Measured 值，两者的差异驱动自适应律
    % =====================================================================
    % 使用上一时刻的控制量 u_filter 进行预测
    x_hat_dot = -Am * x_hat + Bm * u_filter + sigma_hat;
    
    % 欧拉积分更新预测状态
    x_hat_next = x_hat + x_hat_dot * dt;
    
    % =====================================================================
    % 2. 误差计算 (Prediction Error)
    %    x_tilde = x_hat - x_real
    % =====================================================================
    x_tilde = x_hat - Measured;
    
    % =====================================================================
    % 3. 自适应律 (Adaptation Law)
    %    sigma_dot_hat = -Gamma * x_tilde
    %    基于 Lyapunov 稳定性推导，用于快速估计总扰动 sigma
    % =====================================================================
    sigma_dot = -Gamma * x_tilde;
    
    % 更新扰动估计
    sigma_hat_next = sigma_hat + sigma_dot * dt;
    
    % =====================================================================
    % 4. 控制律计算 (Control Law)
    %    目标: 消除扰动 sigma 并跟踪参考信号 Target
    %    u_raw = (Am * Target - sigma_hat) / Bm
    %    (这里假设我们希望闭环系统行为像 dx/dt = -Am*x + Am*Target)
    % =====================================================================
    u_raw = (Am * Target - sigma_hat_next) / Bm;
    
    % =====================================================================
    % 5. 低通滤波器 (Low-Pass Filter) - L1 控制器的关键特征
    %    C(s) = Wc / (s + Wc)
    %    过滤掉高频自适应噪声，仅让低频有效控制信号通过
    % =====================================================================
    u_dot = -Wc * u_filter + Wc * u_raw;
    u_filter_next = u_filter + u_dot * dt;
    
    % =====================================================================
    % 6. 输出限幅与状态更新
    % =====================================================================
    % 物理执行机构限制 (0 ~ 1)
    u_cmd = max(min(u_filter_next, 1), 0);
    
    % 更新 Persistent 变量供下一次计算使用
    x_hat = x_hat_next;
    sigma_hat = sigma_hat_next;
    
    % 注意：这里使用限幅后的 u_cmd 更新 u_filter，
    % 可以在一定程度上防止积分器(滤波器)饱和 (Anti-windup 效应)
    u_filter = u_cmd; 
end

== matlab function EngineBleedAirSystem/Engine Bleed Air System/FAV Actuator ==
  data: cmd_FAV_mA input; theta_FAV output
function theta_FAV = FAV_Actuator(cmd_FAV_mA)
    % =========================================================================
    % FAV 执行机构模型 
    % 
    % 功能: 将电流转换为阀门角度，包含磁滞和动态特性
    % 输入: 
    %   cmd_PRSOV_mA - 控制电流 (0-400mA)
    % 输出: 
    %   theta_PRSOV - 阀门物理角度 (0-90度)
    % =========================================================================
    
    % 仿真步长
    dt = 0.01;

    % 记忆上一次的状态
    persistent Prev_Hys_Angle Prev_Angle is_initialized
    
    % --- 1. 动态初始化 ---
    % 如果是第一次运行，根据当前电流计算初始角度
    if isempty(is_initialized)
        I_start = max(0, min(cmd_FAV_mA, 350));
        
        % 定义基础特性数据
        I_data = [0, 120.0000, 134.3750, 148.7500, 163.1250, 177.5000, ...
              206.2500, 235.0000, 263.7500, 292.5000, 321.2500, 350.0000];
        A_rise_data = [0, 0, 3, 7, 15, 25, 45, 62, 75, 85, 89, 90]; 
        A_fall_data = [0, 0, 10, 25, 40, 55, 75, 85, 89, 90, 90, 90];
        
        % 初始角度
        Prev_Hys_Angle = 0;
        Prev_Angle = Prev_Hys_Angle;
        is_initialized = true;
    end
    
    % --- 2. 输入限幅 ---
    I_safe = max(0, min(cmd_FAV_mA, 350));
    
    % --- 3. 磁滞包络线计算 ---
    I_ref = [0, 120.0000, 134.3750, 148.7500, 163.1250, 177.5000, ...
              206.2500, 235.0000, 263.7500, 292.5000, 321.2500, 350.0000];
    A_rise = [0, 0, 3, 7, 15, 25, 45, 62, 75, 85, 89, 90]; 
    A_fall = [0, 0, 10, 25, 40, 55, 75, 85, 89, 90, 90, 90];
    
    % 计算当前电流对应的上下限
    Limit_Low  = interp1(I_ref, A_rise, I_safe, 'linear', 'extrap');
    Limit_High = interp1(I_ref, A_fall, I_safe, 'linear', 'extrap');
    
    % 限制范围在 0 到 90 度
    Limit_Low  = max(0, min(90, Limit_Low));
    Limit_High = max(0, min(90, Limit_High));
    
    % --- 4. 磁滞逻辑实现 ---
    % 如果电流变化没超过包络线，角度保持不变
    Target_Angle = max(Limit_Low, min(Limit_High, Prev_Hys_Angle));
    Prev_Hys_Angle = Target_Angle;
    
    % --- 5. 惯性环节 (一阶响应) ---
    Tau = 0.1; % 时间常数
    % 使用输入的 dt 计算新角度
    Angle_new = Prev_Angle + (Target_Angle - Prev_Angle) * (dt / (Tau + dt));
    
    % 更新并输出结果
    Prev_Angle = Angle_new;
    theta_FAV = Angle_new;
end

== matlab function EngineBleedAirSystem/Engine Bleed Air System/PRSOV Actuator ==
  data: cmd_PRSOV_mA input; theta_PRSOV output
function theta_PRSOV = PRSOV_Actuator(cmd_PRSOV_mA)
    % =========================================================================
    % PRSOV 执行机构模型 
    % 
    % 功能: 将电流转换为阀门角度，包含磁滞和动态特性
    % 输入: 
    %   cmd_PRSOV_mA - 控制电流 (0-400mA)
    % 输出: 
    %   theta_PRSOV - 阀门物理角度 (0-90度)
    % =========================================================================
    
    % 仿真步长
    dt = 0.01;

    % 记忆上一次的状态
    persistent Prev_Hys_Angle Prev_Angle is_initialized
    
    % --- 1. 动态初始化 ---
    % 如果是第一次运行，根据当前电流计算初始角度
    if isempty(is_initialized)
        I_start = max(0, min(cmd_PRSOV_mA, 400));
        
        % 定义基础特性数据
        I_data = [0, 120.0, 137.5, 155.0, 172.5, 190.0, 225.0, 260.0, 295.0, 330.0, 365.0, 400.0];
        A_rise_data = [0, 0, 3, 7, 15, 25, 45, 62, 75, 85, 89, 90]; 
        A_fall_data = [0, 0, 10, 25, 40, 55, 75, 85, 89, 90, 90, 90];
        
        % 初始角度
        Prev_Hys_Angle = 0;
        Prev_Angle = Prev_Hys_Angle;
        is_initialized = true;
    end
    
    % --- 2. 输入限幅 ---
    I_safe = max(0, min(cmd_PRSOV_mA, 400));
    
    % --- 3. 磁滞包络线计算 ---
    I_ref = [0, 120.0, 137.5, 155.0, 172.5, 190.0, 225.0, 260.0, 295.0, 330.0, 365.0, 400.0];
    A_rise = [0, 0, 3, 7, 15, 25, 45, 62, 75, 85, 89, 90]; 
    A_fall = [0, 0, 10, 25, 40, 55, 75, 85, 89, 90, 90, 90];
    
    % 计算当前电流对应的上下限
    Limit_Low  = interp1(I_ref, A_rise, I_safe, 'linear', 'extrap');
    Limit_High = interp1(I_ref, A_fall, I_safe, 'linear', 'extrap');
    
    % 限制范围在 0 到 90 度
    Limit_Low  = max(0, min(90, Limit_Low));
    Limit_High = max(0, min(90, Limit_High));
    
    % --- 4. 磁滞逻辑实现 ---
    % 如果电流变化没超过包络线，角度保持不变
    Target_Angle = max(Limit_Low, min(Limit_High, Prev_Hys_Angle));
    Prev_Hys_Angle = Target_Angle;
    
    % --- 5. 惯性环节 (一阶响应) ---
    Tau = 0.1; % 时间常数
    % 使用输入的 dt 计算新角度
    Angle_new = Prev_Angle + (Target_Angle - Prev_Angle) * (dt / (Tau + dt));
    
    % 更新并输出结果
    Prev_Angle = Angle_new;
    theta_PRSOV = Angle_new;
end
